simulink model "reset_demo2"  (R2015a)
settings: Solver=ode45  SolverMode=SingleTasking  StartTime=0.0  StopTime=10.0  RelTol=1e-3
settings Model: CovMetricSettings=dwe  CovHtmlReporting=off  covSaveCumulativeToWorkspaceVar=off  CovSaveSingleToWorkspaceVar=off  CovExternalEMLEnable=on  Creator=cbrooks  LastModifiedBy=hbourbou
settings DataIOCC: LimitDataPoints=off  SaveFormat=Dataset
settings DebuggingCC: SFUnexpectedBacktrackingDiag=error  SFNoUnconditionalDefaultTransitionDiag=error
settings HardwareCC: ProdBitPerPointer=64  ProdLargestAtomicFloat=Float  ProdIntDivRoundTo=Zero  ProdEndianess=LittleEndian  ProdHWDeviceType=Specified
settings ModelReferenceCC: PropagateSignalLabelsOutOfModel=on
settings GRTTargetCC: TargetLangStandard=C99 (ISO)  GeneratePreprocessorConditionals=Use local settings

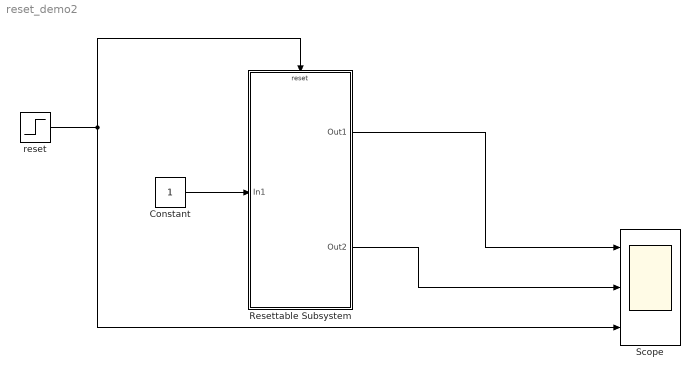
== system reset_demo2 ==
  Constant : Constant  SampleTime=.2
  Resettable Subsystem : Subsystem  TreatAsAtomicUnit=on
  Scope : Scope  NumInputPorts=3
      settings: TimeRange=auto  MaxDataPoints=5000  SaveToWorkspace=off  SaveName=ScopeData  YMin=-3.00000~-3.00000~-0.125  YMax=27.00000~27.00000~1.125  SampleTime=-1
  reset : Step  Time=5  SampleTime=.2
  wires:
  Constant/1 -> Resettable Subsystem/1(In1)
  Resettable Subsystem/1(Out1) -> Scope/1
  Resettable Subsystem/2(Out2) -> Scope/2
  reset/1 -> Scope/3, Resettable Subsystem/Reset

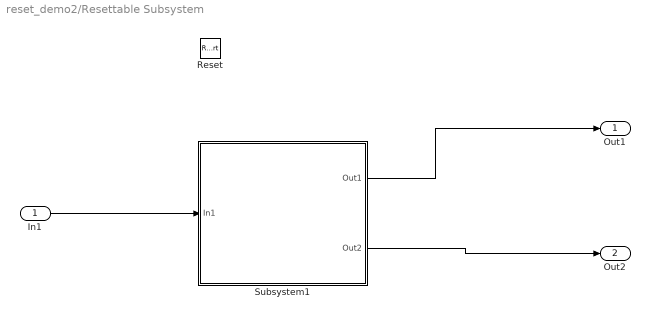
== system reset_demo2/Resettable Subsystem ==
  In1 : Inport
  Reset : ResetPort  DisableCoverage=on  ResetTriggerType=level hold
  Subsystem1 : Subsystem
  Out1 : Outport
  Out2 : Outport  Port=2
  wires:
  In1/1 -> Subsystem1/1(In1)
  Subsystem1/1(Out1) -> Out1/1
  Subsystem1/2(Out2) -> Out2/1

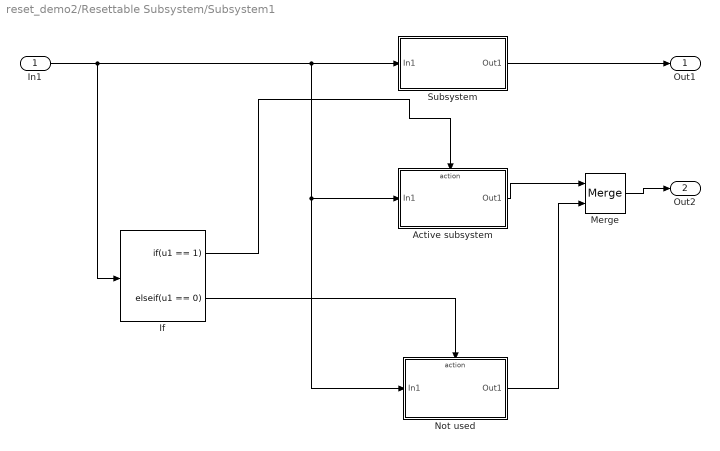
== system reset_demo2/Resettable Subsystem/Subsystem1 ==
  In1 : Inport
  Active subsystem : Subsystem  TreatAsAtomicUnit=on
  If : If  IfExpression=u1 == 1  ElseIfExpressions=u1 == 0  ShowElse=off
  Merge : Merge
  Not used : Subsystem  TreatAsAtomicUnit=on
  Subsystem : Subsystem
  Out1 : Outport
  Out2 : Outport  Port=2
  wires:
  Not used/1(Out1) -> Merge/2
  Merge/1 -> Out2/1
  Subsystem/1(Out1) -> Out1/1
  Active subsystem/1(Out1) -> Merge/1
  If/2 -> Not used/Action
  If/1 -> Active subsystem/Action
  In1/1 -> Subsystem/1(In1), Not used/1(In1), Active subsystem/1(In1), If/1

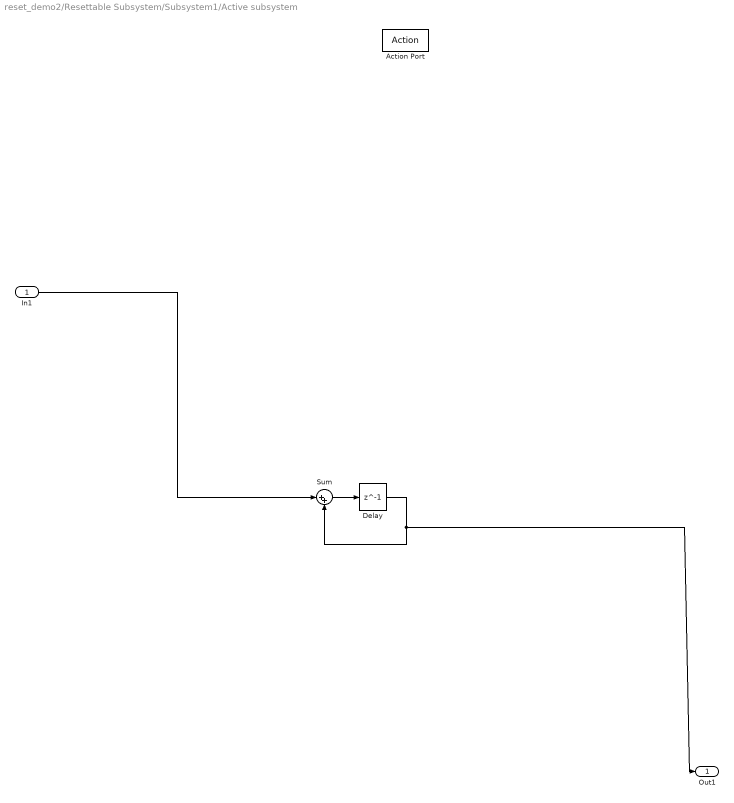
== system reset_demo2/Resettable Subsystem/Subsystem1/Active subsystem ==
  In1 : Inport
  Action Port : ActionPort  ActionType=then
  Delay : Delay  DelayLength=1
  Sum : Sum  Inputs=|++
  Out1 : Outport
  wires:
  Delay/1 -> Out1/1, Sum/2
  In1/1 -> Sum/1
  Sum/1 -> Delay/1

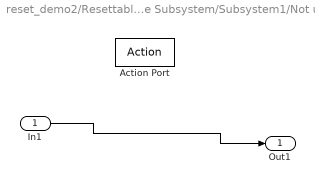
== system reset_demo2/Resettable Subsystem/Subsystem1/Not used ==
  In1 : Inport
  Action Port : ActionPort  ActionType=elseif
  Out1 : Outport
  wires:
  In1/1 -> Out1/1

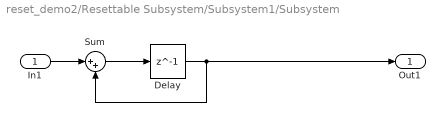
== system reset_demo2/Resettable Subsystem/Subsystem1/Subsystem ==
  In1 : Inport
  Delay : Delay  DelayLength=1
  Sum : Sum  Inputs=|++
  Out1 : Outport
  wires:
  Delay/1 -> Out1/1, Sum/2
  Sum/1 -> Delay/1
  In1/1 -> Sum/1
